simulink model "qr8x8"  (R2018b)
settings: Solver=VariableStepAuto  StartTime=0.0  StopTime=10.0  RelTol=1e-3
libraries: hdlsllib x71, simulink x16, dspmathops x1
(part 1 of 2)
settings Model: Creator=lbai  LastModifiedBy=lbai

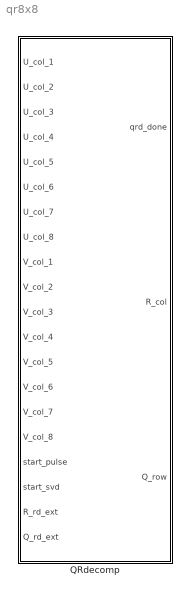
== system qr8x8 ==
  QRdecomp : Subsystem

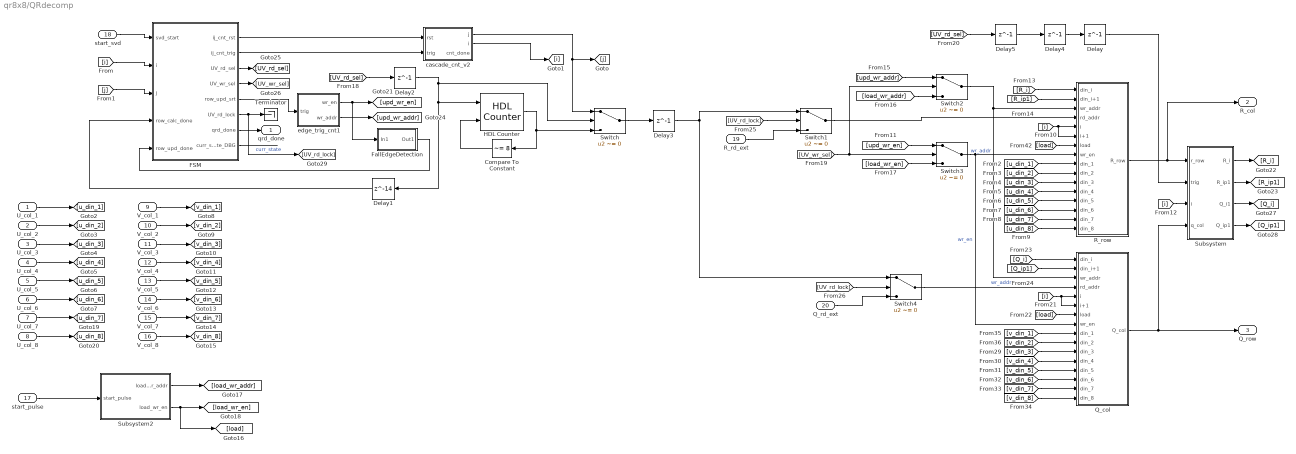
== system qr8x8/QRdecomp ==
  U_col_1 : Inport
  U_col_2 : Inport  Port=2
  U_col_3 : Inport  Port=3
  U_col_4 : Inport  Port=4
  U_col_5 : Inport  Port=5
  U_col_6 : Inport  Port=6
  U_col_7 : Inport  Port=7
  U_col_8 : Inport  Port=8
  V_col_1 : Inport  Port=9
  V_col_2 : Inport  Port=10
  V_col_3 : Inport  Port=11
  V_col_4 : Inport  Port=12
  V_col_5 : Inport  Port=13
  V_col_6 : Inport  Port=14
  V_col_7 : Inport  Port=15
  V_col_8 : Inport  Port=16
  start_pulse : Inport  Port=17
  start_svd : Inport  Port=18
  R_rd_ext : Inport  Port=19
  Q_rd_ext : Inport  Port=20
  Compare To Constant : simulink/Logic and Bit Operations/Compare To Constant  relop=~=  const=8  OutDataTypeStr=boolean
  Delay{,2..5} (5 alike) : Delay  DelayLength=1
  Delay1 : Delay  DelayLength=14
  FSM : MATLAB Function  TreatAsAtomicUnit=on
  FallEdgeDetection : Subsystem
  HDL Counter : hdlsllib/Sources/HDL Counter  CountType=Count limited  CountInit=1  CountStep=1  CountMax=8  CountFromType=Initial value  CountFrom=1  CountResetPort=on  CountLoadPort=off  CountEnbPort=on  CountDirPort=off  CountDataType=Unsigned  CountWordLen=4  CountFracLen=0  CountSampTime=1
      settings: SourceProductBaseCode=HD
  Q_col : Subsystem
  R_row : Subsystem
  Subsystem : Subsystem
  Subsystem2 : Subsystem
  Switch{,1..4} (5 alike) : Switch  Criteria=u2 ~= 0
  Terminator : Terminator
  cascade_cnt_v2 : Subsystem
  edge_trig_cnt1 : Subsystem
  qrd_done : Outport
  R_col : Outport  Port=2
  Q_row : Outport  Port=3
  wires:
  Subsystem2/1(load_wr_addr) -> [load_wr_addr]
  Subsystem2/2(load_wr_en) -> [load], [load_wr_en]
  start_pulse/1 -> Subsystem2/1(start_pulse)
  cascade_cnt_v2/2(i) -> [i]
  [j] -> FSM/3(j)
  FSM/8(curr_state_DBG) -> ?  "curr_state"
  [i] -> FSM/2(i)
  Switch/1 -> Delay3/1
  HDL Counter/1 -> Switch/3, Compare To Constant/1
  FSM/2(ij_cnt_trig) -> cascade_cnt_v2/2(trig)
  [UV_rd_sel] -> Delay2/1
  Compare To Constant/1 -> HDL Counter/2
  [u_din_7] -> R_row/15(din_7)
  start_svd/1 -> FSM/1(svd_start)
  [u_din_6] -> R_row/14(din_6)
  [u_din_4] -> R_row/12(din_4)
  [u_din_8] -> R_row/16(din_8)
  [load] -> R_row/7(load)
  [u_din_1] -> R_row/9(din_1)
  cascade_cnt_v2/1(j) -> Switch/1, [j]
  [u_din_3] -> R_row/11(din_3)
  FSM/1(ij_cnt_rst) -> cascade_cnt_v2/1(rst)
  [u_din_5] -> R_row/13(din_5)
  [u_din_2] -> R_row/10(din_2)
  U_col_1/1 -> [u_din_1]
  U_col_2/1 -> [u_din_2]
  U_col_3/1 -> [u_din_3]
  U_col_4/1 -> [u_din_4]
  U_col_5/1 -> [u_din_5]
  U_col_6/1 -> [u_din_6]
  U_col_7/1 -> [u_din_7]
  U_col_8/1 -> [u_din_8]
  V_col_8/1 -> [v_din_8]
  V_col_7/1 -> [v_din_7]
  V_col_3/1 -> [v_din_3]
  V_col_1/1 -> [v_din_1]
  V_col_4/1 -> [v_din_4]
  V_col_5/1 -> [v_din_5]
  V_col_6/1 -> [v_din_6]
  V_col_2/1 -> [v_din_2]
  [load_wr_en] -> Switch3/3
  [load_wr_addr] -> Switch2/3
  Switch2/1 -> Q_col/3(wr_addr), R_row/3(wr_addr)  "wr_addr"
  Switch3/1 -> Q_col/8(wr_en), R_row/8(wr_en)  "wr_en"
  [UV_wr_sel] -> Switch2/2, Switch3/2
  Switch1/1 -> R_row/4(rd_addr)
  Delay4/1 -> Delay/1
  [i] -> R_row/6(i+1), R_row/5(i)
  [R_i] -> R_row/1(din_i)
  [R_ip1] -> R_row/2(din_i+1)
  R_row/1(R_row) -> R_col/1, Subsystem/1(r_row)
  Delay/1 -> Subsystem/2(trig)
  [i] -> Subsystem/3(i)
  Subsystem/1(R_i) -> [R_i]
  Subsystem/2(R_ip1) -> [R_ip1]
  edge_trig_cnt1/1(wr_en) -> [upd_wr_en], FallEdgeDetection/1(In1)
  FSM/5(row_upd_srt) -> edge_trig_cnt1/1(trig)
  edge_trig_cnt1/2(wr_addr) -> [upd_wr_addr]
  Delay1/1 -> FSM/4(row_calc_done)
  FallEdgeDetection/1(Out1) -> FSM/5(row_upd_done)
  FSM/3(UV_rd_sel) -> [UV_rd_sel]
  FSM/4(UV_wr_sel) -> [UV_wr_sel]
  [upd_wr_en] -> Switch3/1
  [upd_wr_addr] -> Switch2/1
  Delay2/1 -> Delay1/1, HDL Counter/1, Switch/2
  [UV_rd_sel] -> Delay5/1
  Delay5/1 -> Delay4/1
  [v_din_2] -> Q_col/10(din_2)
  [v_din_5] -> Q_col/13(din_5)
  [v_din_3] -> Q_col/11(din_3)
  [v_din_1] -> Q_col/9(din_1)
  [v_din_8] -> Q_col/16(din_8)
  [v_din_4] -> Q_col/12(din_4)
  [v_din_6] -> Q_col/14(din_6)
  [v_din_7] -> Q_col/15(din_7)
  [i] -> Q_col/6(i+1), Q_col/5(i)
  [load] -> Q_col/7(load)
  Q_col/1(Q_col) -> Q_row/1, Subsystem/4(q_col)
  [Q_i] -> Q_col/1(din_i)
  [Q_ip1] -> Q_col/2(din_i+1)
  Subsystem/3(Q_i1) -> [Q_i]
  Subsystem/4(Q_ip1) -> [Q_ip1]
  FSM/7(qrd_done) -> qrd_done/1
  FSM/6(UV_rd_lock) -> Terminator/1, [UV_rd_lock]
  [UV_rd_lock] -> Switch1/2
  [UV_rd_lock] -> Switch4/2
  R_rd_ext/1 -> Switch1/3
  Q_rd_ext/1 -> Switch4/3
  Switch4/1 -> Q_col/4(rd_addr)  "wr_addr"
  Delay3/1 -> Switch4/1, Switch1/1

== system qr8x8/QRdecomp/FallEdgeDetection ==
  In1 : Inport
  Delay : Delay  DelayLength=1
  Logical Operator : Logic  AllPortsSameDT=off  OutDataTypeStr=boolean
  Logical Operator2 : Logic  Operator=NOT  AllPortsSameDT=off  OutDataTypeStr=boolean
  Out1 : Outport
  wires:
  In1/1 -> Logical Operator2/1, Delay/1
  Delay/1 -> Logical Operator/1
  Logical Operator/1 -> Out1/1
  Logical Operator2/1 -> Logical Operator/2

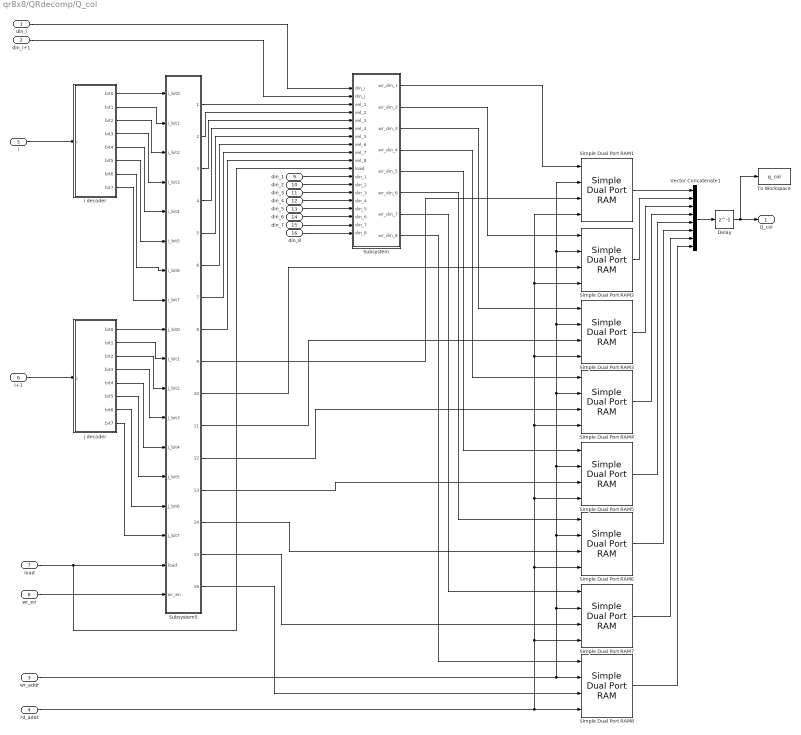
== system qr8x8/QRdecomp/Q_col ==
  din_i : Inport
  din_i+1 : Inport  Port=2
  wr_addr : Inport  Port=3
  rd_addr : Inport  Port=4
  i : Inport  Port=5
  i+1 : Inport  Port=6
  load : Inport  Port=7
  wr_en : Inport  Port=8
  din_1 : Inport  Port=9
  din_2 : Inport  Port=10
  din_3 : Inport  Port=11
  din_4 : Inport  Port=12
  din_5 : Inport  Port=13
  din_6 : Inport  Port=14
  din_7 : Inport  Port=15
  din_8 : Inport  Port=16
  Delay : Delay  DelayLength=1
  Simple Dual Port RAM{1..8} (8 alike) : hdlsllib/HDL RAMs/Simple Dual Port RAM  ram_size=4
      settings: SourceProductName=HDL Coder  SourceProductBaseCode=HD
  Subsystem : Subsystem
  Subsystem5 : Subsystem
  To Workspace : ToWorkspace  VariableName=q_col  SaveFormat=Timeseries  SampleTime=-1
  Vector Concatenate1 : Concatenate  NumInputs=8
  i decoder : MATLAB Function  TreatAsAtomicUnit=on
  j decoder : MATLAB Function  TreatAsAtomicUnit=on
  Q_col : Outport
  wires:
  i+1/1 -> j decoder/1(j)
  Delay/1 -> Q_col/1, To Workspace/1
  Vector Concatenate1/1 -> Delay/1
  Simple Dual Port RAM3/1 -> Vector Concatenate1/3
  Simple Dual Port RAM4/1 -> Vector Concatenate1/4
  Simple Dual Port RAM5/1 -> Vector Concatenate1/5
  Simple Dual Port RAM6/1 -> Vector Concatenate1/6
  Simple Dual Port RAM7/1 -> Vector Concatenate1/7
  Simple Dual Port RAM8/1 -> Vector Concatenate1/8
  i/1 -> i decoder/1(i)
  i decoder/1(bit0) -> Subsystem5/1(i_bit0)
  j decoder/1(bit0) -> Subsystem5/9(j_bit0)
  i decoder/2(bit1) -> Subsystem5/2(i_bit1)
  i decoder/3(bit2) -> Subsystem5/3(i_bit2)
  i decoder/4(bit3) -> Subsystem5/4(i_bit3)
  i decoder/5(bit4) -> Subsystem5/5(i_bit4)
  i decoder/6(bit5) -> Subsystem5/6(i_bit5)
  i decoder/7(bit6) -> Subsystem5/7(i_bit6)
  i decoder/8(bit7) -> Subsystem5/8(i_bit7)
  j decoder/2(bit1) -> Subsystem5/10(j_bit1)
  j decoder/3(bit2) -> Subsystem5/11(j_bit2)
  j decoder/4(bit3) -> Subsystem5/12(j_bit3)
  j decoder/5(bit4) -> Subsystem5/13(j_bit4)
  j decoder/6(bit5) -> Subsystem5/14(j_bit5)
  j decoder/7(bit6) -> Subsystem5/15(j_bit6)
  j decoder/8(bit7) -> Subsystem5/16(j_bit7)
  Subsystem5/9(wr_en_0) -> Simple Dual Port RAM1/3
  Subsystem5/10(wr_en_1) -> Simple Dual Port RAM2/3
  Subsystem5/11(wr_en_2) -> Simple Dual Port RAM3/3
  Subsystem5/12(wr_en_3) -> Simple Dual Port RAM4/3
  Subsystem5/13(wr_en_4) -> Simple Dual Port RAM5/3
  Subsystem5/14(wr_en_5) -> Simple Dual Port RAM6/3
  Subsystem5/15(wr_en_6) -> Simple Dual Port RAM7/3
  Subsystem5/16(wr_en_7) -> Simple Dual Port RAM8/3
  Subsystem5/8(wr_sel_7) -> Subsystem/10(sel_8)
  Subsystem5/7(wr_sel_6) -> Subsystem/9(sel_7)
  Subsystem5/6(wr_sel_5) -> Subsystem/8(sel_6)
  Subsystem5/5(wr_sel_4) -> Subsystem/7(sel_5)
  Subsystem5/4(wr_sel_3) -> Subsystem/6(sel_4)
  Subsystem5/3(wr_sel_2) -> Subsystem/5(sel_3)
  Subsystem5/2(wr_sel_1) -> Subsystem/4(sel_2)
  Subsystem5/1(wr_sel_0) -> Subsystem/3(sel_1)
  din_i/1 -> Subsystem/1(din_i)
  din_i+1/1 -> Subsystem/2("din_j ")
  wr_addr/1 -> Simple Dual Port RAM8/2, Simple Dual Port RAM7/2, Simple Dual Port RAM6/2, Simple Dual Port RAM5/2, Simple Dual Port RAM4/2, Simple Dual Port RAM3/2, Simple Dual Port RAM2/2, Simple Dual Port RAM1/2
  rd_addr/1 -> Simple Dual Port RAM8/4, Simple Dual Port RAM7/4, Simple Dual Port RAM6/4, Simple Dual Port RAM5/4, Simple Dual Port RAM4/4, Simple Dual Port RAM3/4, Simple Dual Port RAM2/4, Simple Dual Port RAM1/4
  Subsystem/1(wr_din_1) -> Simple Dual Port RAM1/1
  Subsystem/2(wr_din_2) -> Simple Dual Port RAM2/1
  Subsystem/3(wr_din_3) -> Simple Dual Port RAM3/1
  Subsystem/4(wr_din_4) -> Simple Dual Port RAM4/1
  Subsystem/5(wr_din_5) -> Simple Dual Port RAM5/1
  Subsystem/6(wr_din_6) -> Simple Dual Port RAM6/1
  Subsystem/7(wr_din_7) -> Simple Dual Port RAM7/1
  Subsystem/8(wr_din_8) -> Simple Dual Port RAM8/1
  wr_en/1 -> Subsystem5/18(wr_en)
  load/1 -> Subsystem/11(load), Subsystem5/17(load)
  din_1/1 -> Subsystem/12(din_1)
  din_2/1 -> Subsystem/13(din_2)
  din_3/1 -> Subsystem/14(din_3)
  din_4/1 -> Subsystem/15(din_4)
  din_5/1 -> Subsystem/16(din_5)
  din_8/1 -> Subsystem/19(din_8)
  din_7/1 -> Subsystem/18(din_7)
  din_6/1 -> Subsystem/17(din_6)
  Simple Dual Port RAM1/1 -> Vector Concatenate1/1
  Simple Dual Port RAM2/1 -> Vector Concatenate1/2

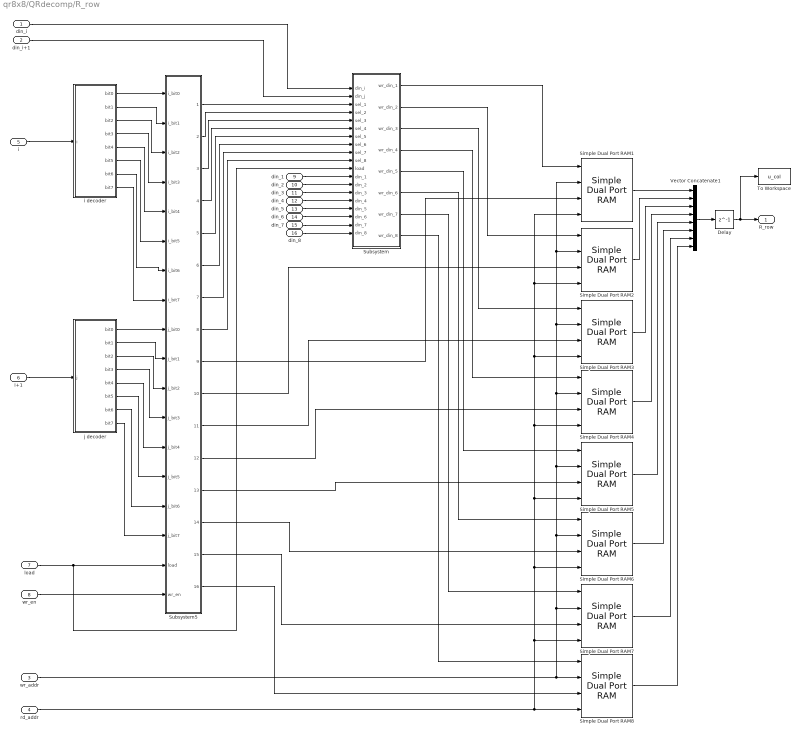
== system qr8x8/QRdecomp/R_row ==
  din_i : Inport
  din_i+1 : Inport  Port=2
  wr_addr : Inport  Port=3
  rd_addr : Inport  Port=4
  i : Inport  Port=5
  i+1 : Inport  Port=6
  load : Inport  Port=7
  wr_en : Inport  Port=8
  din_1 : Inport  Port=9
  din_2 : Inport  Port=10
  din_3 : Inport  Port=11
  din_4 : Inport  Port=12
  din_5 : Inport  Port=13
  din_6 : Inport  Port=14
  din_7 : Inport  Port=15
  din_8 : Inport  Port=16
  Delay : Delay  DelayLength=1
  Simple Dual Port RAM{1..8} (8 alike) : hdlsllib/HDL RAMs/Simple Dual Port RAM  ram_size=4
      settings: SourceProductName=HDL Coder  SourceProductBaseCode=HD
  Subsystem : Subsystem
  Subsystem5 : Subsystem
  To Workspace : ToWorkspace  VariableName=u_col  SaveFormat=Timeseries  SampleTime=-1
  Vector Concatenate1 : Concatenate  NumInputs=8
  i decoder : MATLAB Function  TreatAsAtomicUnit=on
  j decoder : MATLAB Function  TreatAsAtomicUnit=on
  R_row : Outport
  wires:
  Simple Dual Port RAM2/1 -> Vector Concatenate1/2
  Simple Dual Port RAM1/1 -> Vector Concatenate1/1
  din_6/1 -> Subsystem/17(din_6)
  din_7/1 -> Subsystem/18(din_7)
  din_8/1 -> Subsystem/19(din_8)
  din_5/1 -> Subsystem/16(din_5)
  din_4/1 -> Subsystem/15(din_4)
  din_3/1 -> Subsystem/14(din_3)
  din_2/1 -> Subsystem/13(din_2)
  din_1/1 -> Subsystem/12(din_1)
  load/1 -> Subsystem5/17(load), Subsystem/11(load)
  wr_en/1 -> Subsystem5/18(wr_en)
  Subsystem/8(wr_din_8) -> Simple Dual Port RAM8/1
  Subsystem/7(wr_din_7) -> Simple Dual Port RAM7/1
  Subsystem/6(wr_din_6) -> Simple Dual Port RAM6/1
  Subsystem/5(wr_din_5) -> Simple Dual Port RAM5/1
  Subsystem/4(wr_din_4) -> Simple Dual Port RAM4/1
  Subsystem/3(wr_din_3) -> Simple Dual Port RAM3/1
  Subsystem/2(wr_din_2) -> Simple Dual Port RAM2/1
  Subsystem/1(wr_din_1) -> Simple Dual Port RAM1/1
  rd_addr/1 -> Simple Dual Port RAM1/4, Simple Dual Port RAM2/4, Simple Dual Port RAM3/4, Simple Dual Port RAM4/4, Simple Dual Port RAM5/4, Simple Dual Port RAM6/4, Simple Dual Port RAM7/4, Simple Dual Port RAM8/4
  wr_addr/1 -> Simple Dual Port RAM1/2, Simple Dual Port RAM2/2, Simple Dual Port RAM3/2, Simple Dual Port RAM4/2, Simple Dual Port RAM5/2, Simple Dual Port RAM6/2, Simple Dual Port RAM7/2, Simple Dual Port RAM8/2
  din_i+1/1 -> Subsystem/2("din_j ")
  din_i/1 -> Subsystem/1(din_i)
  Subsystem5/1(wr_sel_0) -> Subsystem/3(sel_1)
  Subsystem5/2(wr_sel_1) -> Subsystem/4(sel_2)
  Subsystem5/3(wr_sel_2) -> Subsystem/5(sel_3)
  Subsystem5/4(wr_sel_3) -> Subsystem/6(sel_4)
  Subsystem5/5(wr_sel_4) -> Subsystem/7(sel_5)
  Subsystem5/6(wr_sel_5) -> Subsystem/8(sel_6)
  Subsystem5/7(wr_sel_6) -> Subsystem/9(sel_7)
  Subsystem5/8(wr_sel_7) -> Subsystem/10(sel_8)
  Subsystem5/16(wr_en_7) -> Simple Dual Port RAM8/3
  Subsystem5/15(wr_en_6) -> Simple Dual Port RAM7/3
  Subsystem5/14(wr_en_5) -> Simple Dual Port RAM6/3
  Subsystem5/13(wr_en_4) -> Simple Dual Port RAM5/3
  Subsystem5/12(wr_en_3) -> Simple Dual Port RAM4/3
  Subsystem5/11(wr_en_2) -> Simple Dual Port RAM3/3
  Subsystem5/10(wr_en_1) -> Simple Dual Port RAM2/3
  Subsystem5/9(wr_en_0) -> Simple Dual Port RAM1/3
  j decoder/8(bit7) -> Subsystem5/16(j_bit7)
  j decoder/7(bit6) -> Subsystem5/15(j_bit6)
  j decoder/6(bit5) -> Subsystem5/14(j_bit5)
  j decoder/5(bit4) -> Subsystem5/13(j_bit4)
  j decoder/4(bit3) -> Subsystem5/12(j_bit3)
  j decoder/3(bit2) -> Subsystem5/11(j_bit2)
  j decoder/2(bit1) -> Subsystem5/10(j_bit1)
  i decoder/8(bit7) -> Subsystem5/8(i_bit7)
  i decoder/7(bit6) -> Subsystem5/7(i_bit6)
  i decoder/6(bit5) -> Subsystem5/6(i_bit5)
  i decoder/5(bit4) -> Subsystem5/5(i_bit4)
  i decoder/4(bit3) -> Subsystem5/4(i_bit3)
  i decoder/3(bit2) -> Subsystem5/3(i_bit2)
  i decoder/2(bit1) -> Subsystem5/2(i_bit1)
  j decoder/1(bit0) -> Subsystem5/9(j_bit0)
  i decoder/1(bit0) -> Subsystem5/1(i_bit0)
  i/1 -> i decoder/1(i)
  Simple Dual Port RAM8/1 -> Vector Concatenate1/8
  Simple Dual Port RAM7/1 -> Vector Concatenate1/7
  Simple Dual Port RAM6/1 -> Vector Concatenate1/6
  Simple Dual Port RAM5/1 -> Vector Concatenate1/5
  Simple Dual Port RAM4/1 -> Vector Concatenate1/4
  Simple Dual Port RAM3/1 -> Vector Concatenate1/3
  Vector Concatenate1/1 -> Delay/1
  Delay/1 -> To Workspace/1, R_row/1
  i+1/1 -> j decoder/1(j)

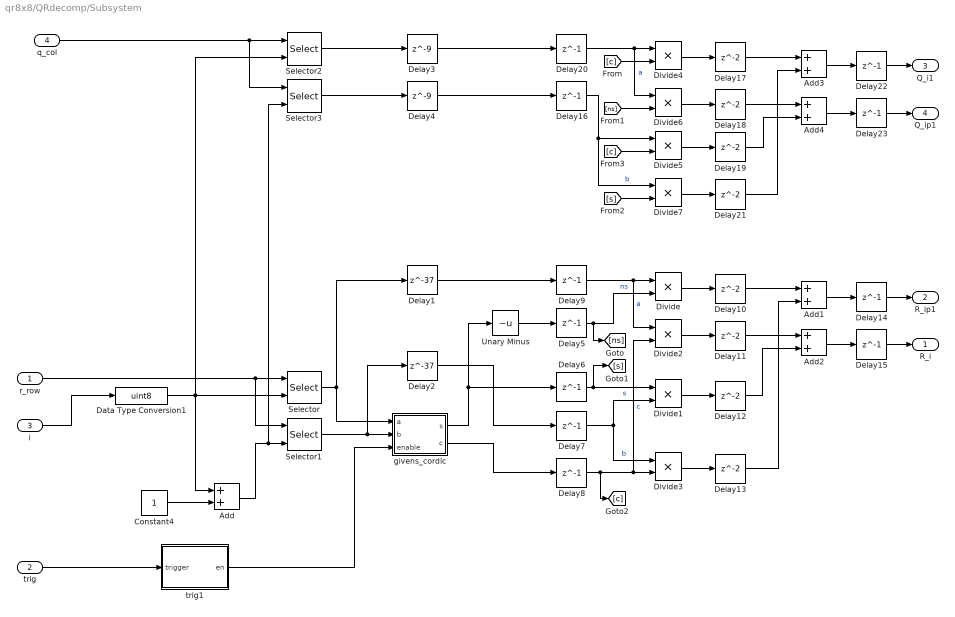
== system qr8x8/QRdecomp/Subsystem ==
  r_row : Inport
  trig : Inport  Port=2
  i : Inport  Port=3
  q_col : Inport  Port=4
  Add : Sum  OutDataTypeStr=Inherit: Same as first input
  Add1 : Sum
  Add2 : Sum
  Add3 : Sum  OutDataTypeStr=fixdt(1,32,30)
  Add4 : Sum  OutDataTypeStr=fixdt(1,32,30)
  Constant4 : Constant  OutDataTypeStr=fixdt(0,1,0)  SampleTime=-1
  Data Type Conversion1 : DataTypeConversion  OutDataTypeStr=uint8
  Delay1 : Delay  DelayLength=37
  Delay{10..13,17..19,21} (8 alike) : Delay
  Delay{5..9,14..16,20,22..23} (11 alike) : Delay  DelayLength=1
  Delay2 : Delay  DelayLength=37
  Delay3 : Delay  DelayLength=9
  Delay4 : Delay  DelayLength=9
  Divide{,1..3} (4 alike) : Product  Inputs=**  OutDataTypeStr=fixdt(1,32,25)  SaturateOnIntegerOverflow=on  RndMeth=Zero
  Divide{4..7} (4 alike) : Product  Inputs=**  OutDataTypeStr=fixdt(1,32,30)  SaturateOnIntegerOverflow=on  RndMeth=Zero
  Selector{,1..3} (4 alike) : Selector  InputPortWidth=8  IndexOptions=Index vector (port)  Indices=[1 3]  OutputSizes=1
  Unary Minus : UnaryMinus
  givens_cordic : Subsystem
  trig1 : Subsystem
  R_i : Outport
  R_ip1 : Outport  Port=2
  Q_i1 : Outport  Port=3
  Q_ip1 : Outport  Port=4
  wires:
  Add1/1 -> Delay14/1
  Delay9/1 -> Divide2/1, Divide/1  "a"
  Unary Minus/1 -> Delay5/1
  Delay8/1 -> [c], Divide2/2, Divide3/2  "c"
  givens_cordic/1(s) -> Unary Minus/1, Delay6/1
  Selector/1 -> givens_cordic/1(a), Delay1/1
  Constant4/1 -> Add/2
  Divide2/1 -> Delay11/1
  Selector1/1 -> givens_cordic/2(b), Delay2/1
  Delay7/1 -> Divide3/1, Divide1/2  "b"
  Divide3/1 -> Delay13/1
  i/1 -> Data Type Conversion1/1
  givens_cordic/2(c) -> Delay8/1
  Delay11/1 -> Add2/1
  trig1/1(en) -> givens_cordic/3(enable)
  r_row/1 -> Selector/1, Selector1/1
  Delay5/1 -> [ns], Divide/2  "ns"
  Delay2/1 -> Delay7/1
  Delay10/1 -> Add1/1
  Delay1/1 -> Delay9/1
  Add2/1 -> Delay15/1
  Delay13/1 -> Add1/2
  Delay12/1 -> Add2/2
  Divide1/1 -> Delay12/1
  Divide/1 -> Delay10/1
  Delay6/1 -> Divide1/1, [s]  "s"
  trig/1 -> trig1/1(trigger)
  Add/1 -> Selector3/2, Selector1/2
  Data Type Conversion1/1 -> Selector2/2, Add/1, Selector/2
  Delay15/1 -> R_i/1
  Delay14/1 -> R_ip1/1
  q_col/1 -> Selector3/1, Selector2/1
  Selector2/1 -> Delay3/1
  Selector3/1 -> Delay4/1
  Delay3/1 -> Delay20/1
  Delay4/1 -> Delay16/1
  Delay20/1 -> Divide6/1, Divide4/1  "a"
  [c] -> Divide4/2
  Delay19/1 -> Add4/2
  Delay21/1 -> Add3/2
  Add4/1 -> Delay23/1
  Delay17/1 -> Add3/1
  Delay18/1 -> Add4/1
  Add3/1 -> Delay22/1
  Divide4/1 -> Delay17/1
  Divide6/1 -> Delay18/1
  Divide5/1 -> Delay19/1
  Divide7/1 -> Delay21/1
  Delay16/1 -> Divide5/1, Divide7/1  "b"
  [s] -> Divide7/2
  [ns] -> Divide6/2
  [c] -> Divide5/2
  Delay22/1 -> Q_i1/1
  Delay23/1 -> Q_ip1/1

== system qr8x8/QRdecomp/Subsystem2 ==
  start_pulse : Inport
  Compare To Constant2 : simulink/Logic and Bit Operations/Compare To Constant  relop===  const=8  OutDataTypeStr=boolean
  Compare To Constant3 : simulink/Logic and Bit Operations/Compare To Constant  relop===  const=0  OutDataTypeStr=boolean
  Constant : Constant  OutDataTypeStr=boolean  SampleTime=-1
  Delay1 : Delay  DelayLength=1
  Delay3 : Delay
  Enabled Resettable Delay : Delay  DelayLength=1  ExternalReset=Level
      settings: InputPortMap=u0,r5
  HDL Counter : hdlsllib/Sources/HDL Counter  CountType=Count limited  CountInit=0  CountStep=1  CountMax=8  CountFromType=Initial value  CountFrom=0  CountResetPort=on  CountLoadPort=off  CountEnbPort=on  CountDirPort=off  CountDataType=Unsigned  CountWordLen=4  CountFracLen=0  CountSampTime=1
      settings: SourceProductBaseCode=HD
  Switch : Switch  Criteria=u2 ~= 0
  load_wr_addr : Outport
  load_wr_en : Outport  Port=2
  wires:
  Compare To Constant3/1 -> HDL Counter/1
  Enabled Resettable Delay/1 -> Delay3/1, HDL Counter/2, Compare To Constant3/1, Switch/3
  Compare To Constant2/1 -> Enabled Resettable Delay/2
  HDL Counter/1 -> Delay1/1, Compare To Constant2/1
  Delay3/1 -> load_wr_en/1
  Constant/1 -> Switch/1
  Switch/1 -> Enabled Resettable Delay/1
  start_pulse/1 -> Switch/2
  Delay1/1 -> load_wr_addr/1

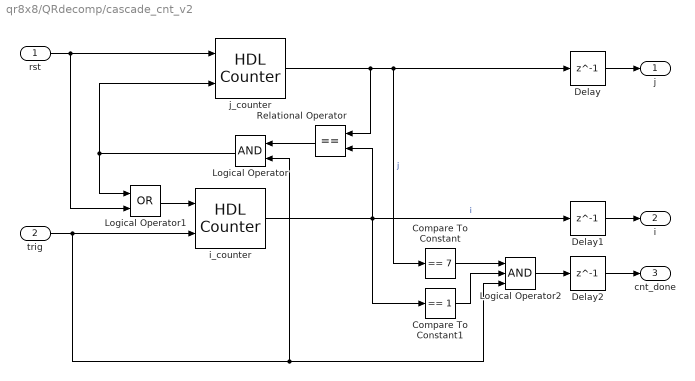
== system qr8x8/QRdecomp/cascade_cnt_v2 ==
  rst : Inport
  trig : Inport  Port=2
  Compare To Constant : simulink/Logic and Bit Operations/Compare To Constant  relop===  const=7  OutDataTypeStr=boolean
  Compare To Constant1 : simulink/Logic and Bit Operations/Compare To Constant  relop===  const=1  OutDataTypeStr=boolean
  Delay : Delay  DelayLength=1
  Delay1 : Delay  DelayLength=1
  Delay2 : Delay  DelayLength=1
  Logical Operator : Logic  AllPortsSameDT=off  OutDataTypeStr=boolean
  Logical Operator1 : Logic  Operator=OR  AllPortsSameDT=off  OutDataTypeStr=boolean
  Logical Operator2 : Logic  Inputs=3  AllPortsSameDT=off  OutDataTypeStr=boolean
  Relational Operator : RelationalOperator  Operator===  OutDataTypeStr=boolean  RndMeth=Nearest
  i_counter : hdlsllib/Sources/HDL Counter  CountType=Count limited  CountInit=7  CountStep=-1  CountMax=1  CountFromType=Initial value  CountFrom=7  CountResetPort=on  CountLoadPort=off  CountEnbPort=on  CountDirPort=off  CountDataType=Unsigned  CountWordLen=4  CountFracLen=0  CountSampTime=1
      settings: SourceProductBaseCode=HD
  j_counter : hdlsllib/Sources/HDL Counter  CountType=Count limited  CountInit=1  CountStep=1  CountMax=7  CountFromType=Initial value  CountFrom=1  CountResetPort=on  CountLoadPort=off  CountEnbPort=on  CountDirPort=off  CountDataType=Unsigned  CountWordLen=4  CountFracLen=0  CountSampTime=1
      settings: SourceProductBaseCode=HD
  j : Outport
  i : Outport  Port=2
  cnt_done : Outport  Port=3
  wires:
  trig/1 -> i_counter/2, Logical Operator/2, Logical Operator2/3
  rst/1 -> Logical Operator1/2, j_counter/1
  j_counter/1 -> Delay/1, Compare To Constant/1, Relational Operator/1  "j"
  i_counter/1 -> Delay1/1, Compare To Constant1/1, Relational Operator/2  "i"
  Relational Operator/1 -> Logical Operator/1
  Logical Operator/1 -> Logical Operator1/1, j_counter/2
  Delay/1 -> j/1
  Delay1/1 -> i/1
  Logical Operator1/1 -> i_counter/1
  Compare To Constant/1 -> Logical Operator2/1
  Compare To Constant1/1 -> Logical Operator2/2
  Logical Operator2/1 -> Delay2/1
  Delay2/1 -> cnt_done/1

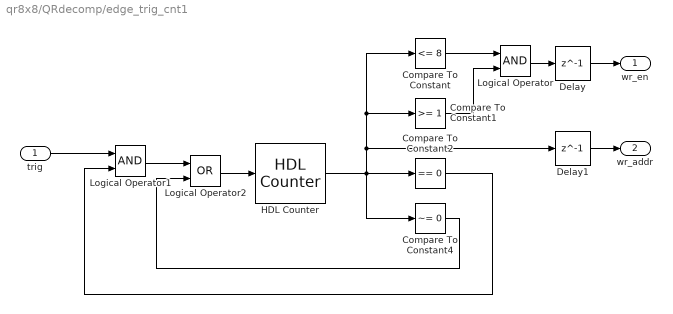
== system qr8x8/QRdecomp/edge_trig_cnt1 ==
  trig : Inport
  Compare To Constant : simulink/Logic and Bit Operations/Compare To Constant  relop=<=  const=8  OutDataTypeStr=boolean
  Compare To Constant1 : simulink/Logic and Bit Operations/Compare To Constant  relop=>=  const=1  OutDataTypeStr=boolean
  Compare To Constant2 : simulink/Logic and Bit Operations/Compare To Constant  relop===  const=0  OutDataTypeStr=boolean
  Compare To Constant4 : simulink/Logic and Bit Operations/Compare To Constant  relop=~=  const=0  OutDataTypeStr=boolean
  Delay : Delay  DelayLength=1
  Delay1 : Delay  DelayLength=1
  HDL Counter : hdlsllib/Sources/HDL Counter  CountType=Count limited  CountInit=0  CountStep=1  CountMax=9  CountFromType=Initial value  CountFrom=0  CountResetPort=off  CountLoadPort=off  CountEnbPort=on  CountDirPort=off  CountDataType=Unsigned  CountWordLen=4  CountFracLen=0  CountSampTime=1
      settings: SourceProductBaseCode=HD
  Logical Operator : Logic  AllPortsSameDT=off  OutDataTypeStr=boolean
  Logical Operator1 : Logic  AllPortsSameDT=off  OutDataTypeStr=boolean
  Logical Operator2 : Logic  Operator=OR  AllPortsSameDT=off  OutDataTypeStr=boolean
  wr_en : Outport
  wr_addr : Outport  Port=2
  wires:
  Delay/1 -> wr_en/1
  Logical Operator2/1 -> HDL Counter/1
  Logical Operator/1 -> Delay/1
  Compare To Constant2/1 -> Logical Operator1/2
  Compare To Constant1/1 -> Logical Operator/2
  trig/1 -> Logical Operator1/1
  Compare To Constant/1 -> Logical Operator/1
  HDL Counter/1 -> Compare To Constant2/1, Compare To Constant4/1, Delay1/1, Compare To Constant1/1, Compare To Constant/1
  Logical Operator1/1 -> Logical Operator2/1
  Compare To Constant4/1 -> Logical Operator2/2
  Delay1/1 -> wr_addr/1

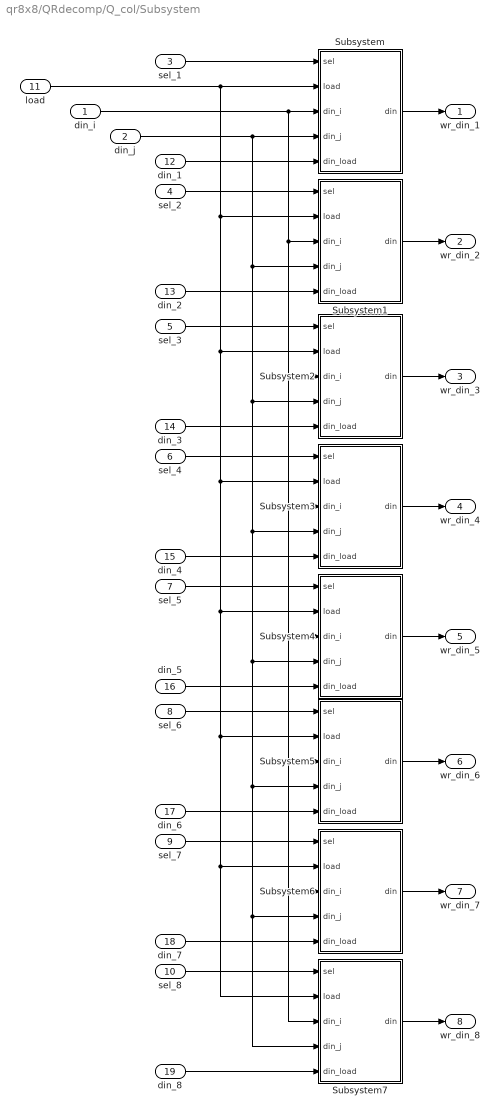
== system qr8x8/QRdecomp/Q_col/Subsystem ==
  din_i : Inport
  "din_j " : Inport  Port=2
  sel_1 : Inport  Port=3
  sel_2 : Inport  Port=4
  sel_3 : Inport  Port=5
  sel_4 : Inport  Port=6
  sel_5 : Inport  Port=7
  sel_6 : Inport  Port=8
  sel_7 : Inport  Port=9
  sel_8 : Inport  Port=10
  load : Inport  Port=11
  din_1 : Inport  Port=12
  din_2 : Inport  Port=13
  din_3 : Inport  Port=14
  din_4 : Inport  Port=15
  din_5 : Inport  Port=16
  din_6 : Inport  Port=17
  din_7 : Inport  Port=18
  din_8 : Inport  Port=19
  Subsystem : Subsystem
  Subsystem1 : Subsystem
  Subsystem2 : Subsystem
  Subsystem3 : Subsystem
  Subsystem4 : Subsystem
  Subsystem5 : Subsystem
  Subsystem6 : Subsystem
  Subsystem7 : Subsystem
  wr_din_1 : Outport
  wr_din_2 : Outport  Port=2
  wr_din_3 : Outport  Port=3
  wr_din_4 : Outport  Port=4
  wr_din_5 : Outport  Port=5
  wr_din_6 : Outport  Port=6
  wr_din_7 : Outport  Port=7
  wr_din_8 : Outport  Port=8
  wires:
  sel_1/1 -> Subsystem/1(sel)
  Subsystem/1(din) -> wr_din_1/1
  "din_j "/1 -> Subsystem/4("din_j "), Subsystem1/4("din_j "), Subsystem2/4("din_j "), Subsystem3/4("din_j "), Subsystem4/4("din_j "), Subsystem5/4("din_j "), Subsystem7/4("din_j "), Subsystem6/4("din_j ")
  Subsystem1/1(din) -> wr_din_2/1
  Subsystem2/1(din) -> wr_din_3/1
  Subsystem3/1(din) -> wr_din_4/1
  Subsystem4/1(din) -> wr_din_5/1
  Subsystem5/1(din) -> wr_din_6/1
  Subsystem6/1(din) -> wr_din_7/1
  Subsystem7/1(din) -> wr_din_8/1
  sel_2/1 -> Subsystem1/1(sel)
  sel_3/1 -> Subsystem2/1(sel)
  sel_4/1 -> Subsystem3/1(sel)
  sel_5/1 -> Subsystem4/1(sel)
  sel_8/1 -> Subsystem7/1(sel)
  load/1 -> Subsystem7/2(load), Subsystem6/2(load), Subsystem5/2(load), Subsystem4/2(load), Subsystem3/2(load), Subsystem2/2(load), Subsystem1/2(load), Subsystem/2(load)
  din_1/1 -> Subsystem/5(din_load)
  din_2/1 -> Subsystem1/5(din_load)
  din_i/1 -> Subsystem/3(din_i), Subsystem2/3(din_i), Subsystem3/3(din_i), Subsystem5/3(din_i), Subsystem7/3(din_i), Subsystem6/3(din_i), Subsystem4/3(din_i), Subsystem1/3(din_i)
  sel_6/1 -> Subsystem5/1(sel)
  sel_7/1 -> Subsystem6/1(sel)
  din_3/1 -> Subsystem2/5(din_load)
  din_4/1 -> Subsystem3/5(din_load)
  din_5/1 -> Subsystem4/5(din_load)
  din_6/1 -> Subsystem5/5(din_load)
  din_7/1 -> Subsystem6/5(din_load)
  din_8/1 -> Subsystem7/5(din_load)

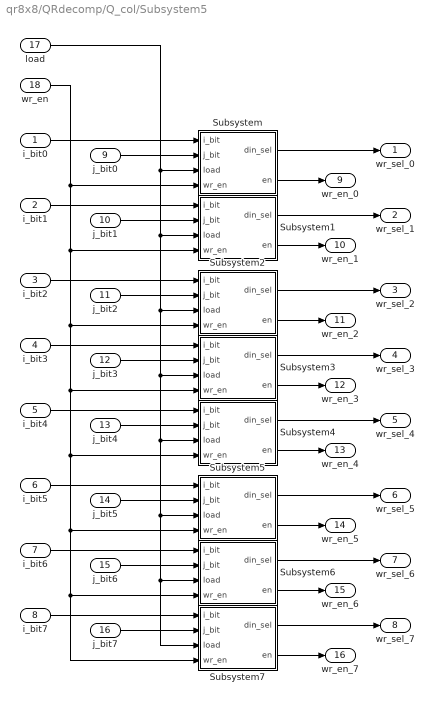
== system qr8x8/QRdecomp/Q_col/Subsystem5 ==
  i_bit0 : Inport
  i_bit1 : Inport  Port=2
  i_bit2 : Inport  Port=3
  i_bit3 : Inport  Port=4
  i_bit4 : Inport  Port=5
  i_bit5 : Inport  Port=6
  i_bit6 : Inport  Port=7
  i_bit7 : Inport  Port=8
  j_bit0 : Inport  Port=9
  j_bit1 : Inport  Port=10
  j_bit2 : Inport  Port=11
  j_bit3 : Inport  Port=12
  j_bit4 : Inport  Port=13
  j_bit5 : Inport  Port=14
  j_bit6 : Inport  Port=15
  j_bit7 : Inport  Port=16
  load : Inport  Port=17
  wr_en : Inport  Port=18
  Subsystem : Subsystem
  Subsystem1 : Subsystem
  Subsystem2 : Subsystem
  Subsystem3 : Subsystem
  Subsystem4 : Subsystem
  Subsystem5 : Subsystem
  Subsystem6 : Subsystem
  Subsystem7 : Subsystem
  wr_sel_0 : Outport
  wr_sel_1 : Outport  Port=2
  wr_sel_2 : Outport  Port=3
  wr_sel_3 : Outport  Port=4
  wr_sel_4 : Outport  Port=5
  wr_sel_5 : Outport  Port=6
  wr_sel_6 : Outport  Port=7
  wr_sel_7 : Outport  Port=8
  wr_en_0 : Outport  Port=9
  wr_en_1 : Outport  Port=10
  wr_en_2 : Outport  Port=11
  wr_en_3 : Outport  Port=12
  wr_en_4 : Outport  Port=13
  wr_en_5 : Outport  Port=14
  wr_en_6 : Outport  Port=15
  wr_en_7 : Outport  Port=16
  wires:
  i_bit1/1 -> Subsystem1/1(i_bit)
  Subsystem4/1(din_sel) -> wr_sel_4/1
  j_bit0/1 -> Subsystem/2(j_bit)
  Subsystem3/2(en) -> wr_en_3/1
  i_bit0/1 -> Subsystem/1(i_bit)
  Subsystem/2(en) -> wr_en_0/1
  i_bit3/1 -> Subsystem3/1(i_bit)
  Subsystem/1(din_sel) -> wr_sel_0/1
  Subsystem2/1(din_sel) -> wr_sel_2/1
  j_bit2/1 -> Subsystem2/2(j_bit)
  j_bit3/1 -> Subsystem3/2(j_bit)
  Subsystem2/2(en) -> wr_en_2/1
  Subsystem3/1(din_sel) -> wr_sel_3/1
  j_bit4/1 -> Subsystem4/2(j_bit)
  Subsystem1/1(din_sel) -> wr_sel_1/1
  Subsystem4/2(en) -> wr_en_4/1
  i_bit4/1 -> Subsystem4/1(i_bit)
  Subsystem1/2(en) -> wr_en_1/1
  i_bit5/1 -> Subsystem5/1(i_bit)
  j_bit5/1 -> Subsystem5/2(j_bit)
  i_bit7/1 -> Subsystem7/1(i_bit)
  j_bit7/1 -> Subsystem7/2(j_bit)
  Subsystem5/1(din_sel) -> wr_sel_5/1
  Subsystem5/2(en) -> wr_en_5/1
  Subsystem6/1(din_sel) -> wr_sel_6/1
  Subsystem6/2(en) -> wr_en_6/1
  Subsystem7/1(din_sel) -> wr_sel_7/1
  Subsystem7/2(en) -> wr_en_7/1
  j_bit1/1 -> Subsystem1/2(j_bit)
  i_bit2/1 -> Subsystem2/1(i_bit)
  i_bit6/1 -> Subsystem6/1(i_bit)
  j_bit6/1 -> Subsystem6/2(j_bit)
  load/1 -> Subsystem1/3(load), Subsystem2/3(load), Subsystem3/3(load), Subsystem4/3(load), Subsystem5/3(load), Subsystem7/3(load), Subsystem6/3(load), Subsystem/3(load)
  wr_en/1 -> Subsystem1/4(wr_en), Subsystem2/4(wr_en), Subsystem3/4(wr_en), Subsystem4/4(wr_en), Subsystem5/4(wr_en), Subsystem7/4(wr_en), Subsystem6/4(wr_en), Subsystem/4(wr_en)

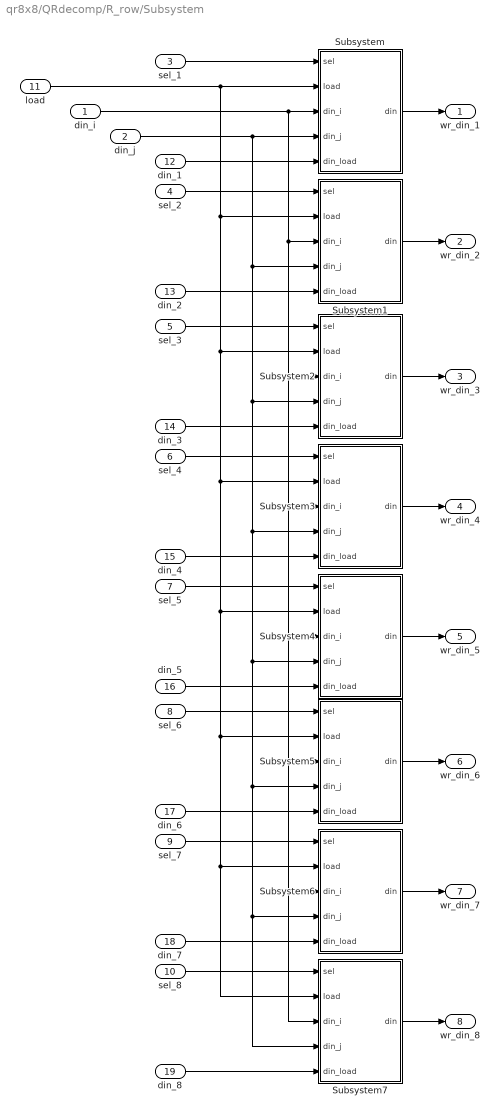
== system qr8x8/QRdecomp/R_row/Subsystem ==
  din_i : Inport
  "din_j " : Inport  Port=2
  sel_1 : Inport  Port=3
  sel_2 : Inport  Port=4
  sel_3 : Inport  Port=5
  sel_4 : Inport  Port=6
  sel_5 : Inport  Port=7
  sel_6 : Inport  Port=8
  sel_7 : Inport  Port=9
  sel_8 : Inport  Port=10
  load : Inport  Port=11
  din_1 : Inport  Port=12
  din_2 : Inport  Port=13
  din_3 : Inport  Port=14
  din_4 : Inport  Port=15
  din_5 : Inport  Port=16
  din_6 : Inport  Port=17
  din_7 : Inport  Port=18
  din_8 : Inport  Port=19
  Subsystem : Subsystem
  Subsystem1 : Subsystem
  Subsystem2 : Subsystem
  Subsystem3 : Subsystem
  Subsystem4 : Subsystem
  Subsystem5 : Subsystem
  Subsystem6 : Subsystem
  Subsystem7 : Subsystem
  wr_din_1 : Outport
  wr_din_2 : Outport  Port=2
  wr_din_3 : Outport  Port=3
  wr_din_4 : Outport  Port=4
  wr_din_5 : Outport  Port=5
  wr_din_6 : Outport  Port=6
  wr_din_7 : Outport  Port=7
  wr_din_8 : Outport  Port=8
  wires:
  din_8/1 -> Subsystem7/5(din_load)
  din_7/1 -> Subsystem6/5(din_load)
  din_6/1 -> Subsystem5/5(din_load)
  din_5/1 -> Subsystem4/5(din_load)
  din_4/1 -> Subsystem3/5(din_load)
  din_3/1 -> Subsystem2/5(din_load)
  sel_7/1 -> Subsystem6/1(sel)
  sel_6/1 -> Subsystem5/1(sel)
  din_i/1 -> Subsystem1/3(din_i), Subsystem4/3(din_i), Subsystem6/3(din_i), Subsystem7/3(din_i), Subsystem5/3(din_i), Subsystem3/3(din_i), Subsystem2/3(din_i), Subsystem/3(din_i)
  din_2/1 -> Subsystem1/5(din_load)
  din_1/1 -> Subsystem/5(din_load)
  load/1 -> Subsystem/2(load), Subsystem1/2(load), Subsystem2/2(load), Subsystem3/2(load), Subsystem4/2(load), Subsystem5/2(load), Subsystem6/2(load), Subsystem7/2(load)
  sel_8/1 -> Subsystem7/1(sel)
  sel_5/1 -> Subsystem4/1(sel)
  sel_4/1 -> Subsystem3/1(sel)
  sel_3/1 -> Subsystem2/1(sel)
  sel_2/1 -> Subsystem1/1(sel)
  Subsystem7/1(din) -> wr_din_8/1
  Subsystem6/1(din) -> wr_din_7/1
  Subsystem5/1(din) -> wr_din_6/1
  Subsystem4/1(din) -> wr_din_5/1
  Subsystem3/1(din) -> wr_din_4/1
  Subsystem2/1(din) -> wr_din_3/1
  Subsystem1/1(din) -> wr_din_2/1
  "din_j "/1 -> Subsystem6/4("din_j "), Subsystem7/4("din_j "), Subsystem5/4("din_j "), Subsystem4/4("din_j "), Subsystem3/4("din_j "), Subsystem2/4("din_j "), Subsystem1/4("din_j "), Subsystem/4("din_j ")
  Subsystem/1(din) -> wr_din_1/1
  sel_1/1 -> Subsystem/1(sel)

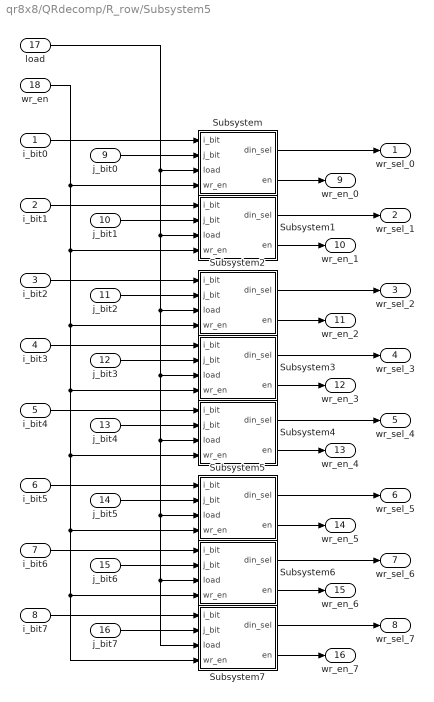
== system qr8x8/QRdecomp/R_row/Subsystem5 ==
  i_bit0 : Inport
  i_bit1 : Inport  Port=2
  i_bit2 : Inport  Port=3
  i_bit3 : Inport  Port=4
  i_bit4 : Inport  Port=5
  i_bit5 : Inport  Port=6
  i_bit6 : Inport  Port=7
  i_bit7 : Inport  Port=8
  j_bit0 : Inport  Port=9
  j_bit1 : Inport  Port=10
  j_bit2 : Inport  Port=11
  j_bit3 : Inport  Port=12
  j_bit4 : Inport  Port=13
  j_bit5 : Inport  Port=14
  j_bit6 : Inport  Port=15
  j_bit7 : Inport  Port=16
  load : Inport  Port=17
  wr_en : Inport  Port=18
  Subsystem : Subsystem
  Subsystem1 : Subsystem
  Subsystem2 : Subsystem
  Subsystem3 : Subsystem
  Subsystem4 : Subsystem
  Subsystem5 : Subsystem
  Subsystem6 : Subsystem
  Subsystem7 : Subsystem
  wr_sel_0 : Outport
  wr_sel_1 : Outport  Port=2
  wr_sel_2 : Outport  Port=3
  wr_sel_3 : Outport  Port=4
  wr_sel_4 : Outport  Port=5
  wr_sel_5 : Outport  Port=6
  wr_sel_6 : Outport  Port=7
  wr_sel_7 : Outport  Port=8
  wr_en_0 : Outport  Port=9
  wr_en_1 : Outport  Port=10
  wr_en_2 : Outport  Port=11
  wr_en_3 : Outport  Port=12
  wr_en_4 : Outport  Port=13
  wr_en_5 : Outport  Port=14
  wr_en_6 : Outport  Port=15
  wr_en_7 : Outport  Port=16
  wires:
  wr_en/1 -> Subsystem/4(wr_en), Subsystem6/4(wr_en), Subsystem7/4(wr_en), Subsystem5/4(wr_en), Subsystem4/4(wr_en), Subsystem3/4(wr_en), Subsystem2/4(wr_en), Subsystem1/4(wr_en)
  load/1 -> Subsystem/3(load), Subsystem6/3(load), Subsystem7/3(load), Subsystem5/3(load), Subsystem4/3(load), Subsystem3/3(load), Subsystem2/3(load), Subsystem1/3(load)
  j_bit6/1 -> Subsystem6/2(j_bit)
  i_bit6/1 -> Subsystem6/1(i_bit)
  i_bit2/1 -> Subsystem2/1(i_bit)
  j_bit1/1 -> Subsystem1/2(j_bit)
  Subsystem7/2(en) -> wr_en_7/1
  Subsystem7/1(din_sel) -> wr_sel_7/1
  Subsystem6/2(en) -> wr_en_6/1
  Subsystem6/1(din_sel) -> wr_sel_6/1
  Subsystem5/2(en) -> wr_en_5/1
  Subsystem5/1(din_sel) -> wr_sel_5/1
  j_bit7/1 -> Subsystem7/2(j_bit)
  i_bit7/1 -> Subsystem7/1(i_bit)
  j_bit5/1 -> Subsystem5/2(j_bit)
  i_bit5/1 -> Subsystem5/1(i_bit)
  Subsystem1/2(en) -> wr_en_1/1
  i_bit4/1 -> Subsystem4/1(i_bit)
  Subsystem4/2(en) -> wr_en_4/1
  Subsystem1/1(din_sel) -> wr_sel_1/1
  j_bit4/1 -> Subsystem4/2(j_bit)
  Subsystem3/1(din_sel) -> wr_sel_3/1
  Subsystem2/2(en) -> wr_en_2/1
  j_bit3/1 -> Subsystem3/2(j_bit)
  j_bit2/1 -> Subsystem2/2(j_bit)
  Subsystem2/1(din_sel) -> wr_sel_2/1
  Subsystem/1(din_sel) -> wr_sel_0/1
  i_bit3/1 -> Subsystem3/1(i_bit)
  Subsystem/2(en) -> wr_en_0/1
  i_bit0/1 -> Subsystem/1(i_bit)
  Subsystem3/2(en) -> wr_en_3/1
  j_bit0/1 -> Subsystem/2(j_bit)
  Subsystem4/1(din_sel) -> wr_sel_4/1
  i_bit1/1 -> Subsystem1/1(i_bit)

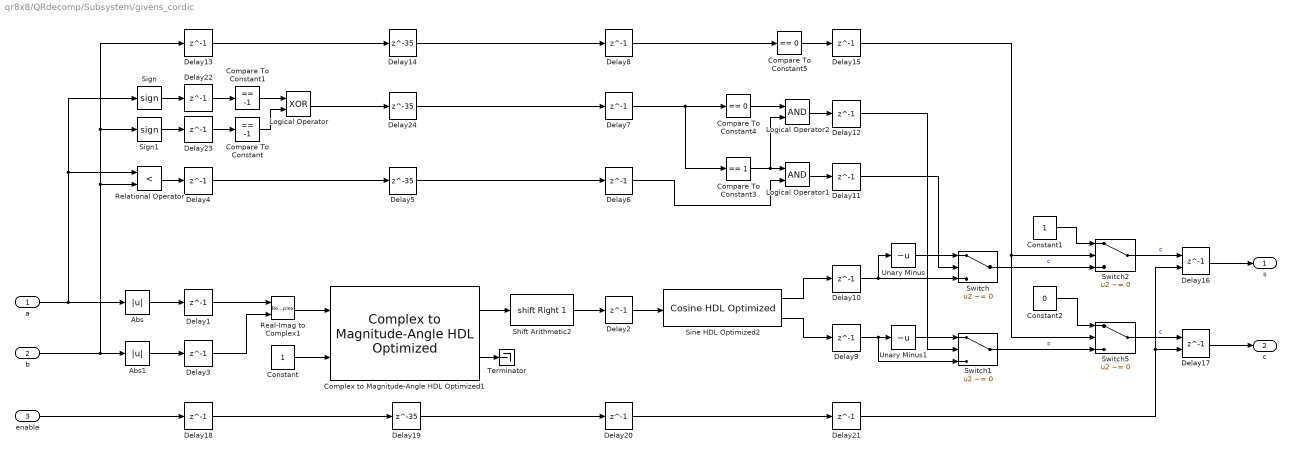
== system qr8x8/QRdecomp/Subsystem/givens_cordic ==
  a : Inport
  b : Inport  Port=2
  enable : Inport  Port=3
  Abs : Abs
  Abs1 : Abs
  Compare To Constant : simulink/Logic and Bit Operations/Compare To Constant  relop===  const=-1  OutDataTypeStr=boolean
  Compare To Constant1 : simulink/Logic and Bit Operations/Compare To Constant  relop===  const=-1  OutDataTypeStr=boolean
  Compare To Constant3 : simulink/Logic and Bit Operations/Compare To Constant  relop===  const=1  OutDataTypeStr=boolean
  Compare To Constant4 : simulink/Logic and Bit Operations/Compare To Constant  relop===  const=0  OutDataTypeStr=boolean
  Compare To Constant5 : simulink/Logic and Bit Operations/Compare To Constant  relop===  const=0  OutDataTypeStr=boolean
  Complex to Magnitude-Angle HDL Optimized1 : dspmathops/Complex to Magnitude-Angle HDL Optimized  NumIterationsSource=Auto  NumIterations=8  OutputFormat=Angle  AngleFormat=Normalized  ScaleOutput=on  SimulateUsing=Code generation
      settings: SourceProductName=DSP System Toolbox  SourceProductBaseCode=DS
  Constant : Constant  OutDataTypeStr=boolean  SampleTime=-1
  Constant1 : Constant  OutDataTypeStr=fixdt(1,32,30)  SampleTime=-1
  Constant2 : Constant  Value=0  OutDataTypeStr=fixdt(1,32,30)  SampleTime=-1
  Delay{1..4,6..13,15,18,20..23} (18 alike) : Delay  DelayLength=1
  Delay{5,14,19,24} (4 alike) : Delay  DelayLength=35
  Delay16 : Delay  DelayLength=1  ShowEnablePort=on
      settings: InputPortMap=u0,e6
  Delay17 : Delay  DelayLength=1  ShowEnablePort=on
      settings: InputPortMap=u0,e6
  Logical Operator : Logic  Operator=XOR  AllPortsSameDT=off  OutDataTypeStr=boolean
  Logical Operator1 : Logic  AllPortsSameDT=off  OutDataTypeStr=boolean
  Logical Operator2 : Logic  AllPortsSameDT=off  OutDataTypeStr=boolean
  Real-Imag to Complex1 : RealImagToComplex
  Relational Operator : RelationalOperator  Operator=<  OutDataTypeStr=boolean  RndMeth=Nearest
  Shift Arithmetic2 : ArithShift  BitShiftNumber=1  BitShiftDirection=Right
  Sign : Signum
  Sign1 : Signum
  Sine HDL Optimized2 : hdlsllib/Lookup Tables/Cosine HDL Optimized  OutputFormula=sin(2*pi*u) and cos(2*pi*u)  NumDataPoints=512  TableDataTypeStr=fixdt(1,32,30)  SimulateLUTROMDelay=off
      settings: SourceProductName=HDL Coder  SourceProductBaseCode=HD
  Switch{,1..2,5} (4 alike) : Switch  Criteria=u2 ~= 0
  Terminator : Terminator
  Unary Minus : UnaryMinus
  Unary Minus1 : UnaryMinus
  s : Outport
  c : Outport  Port=2
  wires:
  Delay2/1 -> Sine HDL Optimized2/1
  Shift Arithmetic2/1 -> Delay2/1
  Real-Imag to Complex1/1 -> Complex to Magnitude-Angle HDL Optimized1/1
  Complex to Magnitude-Angle HDL Optimized1/2 -> Terminator/1
  Constant/1 -> Complex to Magnitude-Angle HDL Optimized1/2
  Complex to Magnitude-Angle HDL Optimized1/1 -> Shift Arithmetic2/1
  Sine HDL Optimized2/1 -> Delay10/1
  Sine HDL Optimized2/2 -> Delay9/1
  Abs/1 -> Delay1/1
  Abs1/1 -> Delay3/1
  Compare To Constant3/1 -> Logical Operator2/2, Logical Operator1/1
  Delay23/1 -> Compare To Constant/1
  Delay13/1 -> Delay14/1
  Sign/1 -> Delay22/1
  Compare To Constant4/1 -> Logical Operator2/1
  Compare To Constant1/1 -> Logical Operator/1
  Delay22/1 -> Compare To Constant1/1
  Compare To Constant/1 -> Logical Operator/2
  Logical Operator/1 -> Delay24/1
  Sign1/1 -> Delay23/1
  Delay16/1 -> s/1
  Switch5/1 -> Delay17/1  "c"
  Switch/1 -> Switch2/3  "c"
  Constant2/1 -> Switch5/1
  Constant1/1 -> Switch2/1
  Switch1/1 -> Switch5/3  "s"
  Switch2/1 -> Delay16/1  "c"
  Delay17/1 -> c/1
  Delay1/1 -> Real-Imag to Complex1/1
  Delay3/1 -> Real-Imag to Complex1/2
  b/1 -> Relational Operator/2, Delay13/1, Sign1/1, Abs1/1
  a/1 -> Relational Operator/1, Sign/1, Abs/1
  Relational Operator/1 -> Delay4/1
  Delay4/1 -> Delay5/1
  Delay5/1 -> Delay6/1
  Delay24/1 -> Delay7/1
  Delay14/1 -> Delay8/1
  Delay7/1 -> Compare To Constant3/1, Compare To Constant4/1
  Delay6/1 -> Logical Operator1/2
  Unary Minus/1 -> Switch/1
  Unary Minus1/1 -> Switch1/1
  Logical Operator1/1 -> Delay11/1
  Logical Operator2/1 -> Delay12/1
  Delay8/1 -> Compare To Constant5/1
  Compare To Constant5/1 -> Delay15/1
  Delay19/1 -> Delay20/1
  Delay21/1 -> Delay17/2, Delay16/2
  Delay20/1 -> Delay21/1
  Delay18/1 -> Delay19/1
  enable/1 -> Delay18/1
  Delay9/1 -> Switch1/3, Unary Minus1/1
  Delay10/1 -> Unary Minus/1, Switch/3
  Delay11/1 -> Switch/2
  Delay12/1 -> Switch1/2
  Delay15/1 -> Switch5/2, Switch2/2

== system qr8x8/QRdecomp/Subsystem/trig1 ==
  trigger : Inport
  Compare To Constant2 : simulink/Logic and Bit Operations/Compare To Constant  relop===  const=2  OutDataTypeStr=boolean
  Compare To Constant3 : simulink/Logic and Bit Operations/Compare To Constant  relop===  const=0  OutDataTypeStr=boolean
  Constant : Constant  OutDataTypeStr=boolean  SampleTime=-1
  Enabled Resettable Delay : Delay  DelayLength=1  ExternalReset=Level
      settings: InputPortMap=u0,r5
  HDL Counter : hdlsllib/Sources/HDL Counter  CountType=Count limited  CountInit=0  CountStep=1  CountMax=2  CountFromType=Initial value  CountFrom=0  CountResetPort=on  CountLoadPort=off  CountEnbPort=on  CountDirPort=off  CountDataType=Unsigned  CountWordLen=4  CountFracLen=0  CountSampTime=1
      settings: SourceProductBaseCode=HD
  Switch : Switch  Criteria=u2 ~= 0
  en : Outport
  wires:
  Compare To Constant2/1 -> Enabled Resettable Delay/2
  Enabled Resettable Delay/1 -> Switch/3, Compare To Constant3/1, HDL Counter/2, en/1
  Compare To Constant3/1 -> HDL Counter/1
  HDL Counter/1 -> Compare To Constant2/1
  Switch/1 -> Enabled Resettable Delay/1
  Constant/1 -> Switch/1
  trigger/1 -> Switch/2

== system qr8x8/QRdecomp/Q_col/Subsystem/Subsystem ==
  sel : Inport
  load : Inport  Port=2
  din_i : Inport  Port=3
  "din_j " : Inport  Port=4
  din_load : Inport  Port=5
  Bit Slice : hdlsllib/Logic and Bit Operations/Bit Slice  lidx=1  ridx=1
  Bit Slice1 : hdlsllib/Logic and Bit Operations/Bit Slice  lidx=0  ridx=0
  Constant : Constant  Value=0  OutDataTypeStr=fixdt(1,32,25)  SampleTime=-1
  Logical Operator : Logic  Operator=XOR  AllPortsSameDT=off  OutDataTypeStr=boolean
  Switch : Switch  Criteria=u2 ~= 0
  Switch1 : Switch  Criteria=u2 ~= 0
  Switch2 : Switch  Criteria=u2 ~= 0
  din : Outport
  wires:
  Constant/1 -> Switch2/3
  Logical Operator/1 -> Switch2/2
  sel/1 -> Bit Slice1/1, Bit Slice/1
  din_i/1 -> Switch/1
  Bit Slice1/1 -> Switch/2, Logical Operator/2
  Bit Slice/1 -> Logical Operator/1
  Switch/1 -> Switch2/1
  "din_j "/1 -> Switch/3
  Switch1/1 -> din/1
  din_load/1 -> Switch1/1
  load/1 -> Switch1/2
  Switch2/1 -> Switch1/3

== system qr8x8/QRdecomp/Q_col/Subsystem/Subsystem1 ==
  sel : Inport
  load : Inport  Port=2
  din_i : Inport  Port=3
  "din_j " : Inport  Port=4
  din_load : Inport  Port=5
  Bit Slice : hdlsllib/Logic and Bit Operations/Bit Slice  lidx=1  ridx=1
  Bit Slice1 : hdlsllib/Logic and Bit Operations/Bit Slice  lidx=0  ridx=0
  Constant : Constant  Value=0  OutDataTypeStr=fixdt(1,32,25)  SampleTime=-1
  Logical Operator : Logic  Operator=XOR  AllPortsSameDT=off  OutDataTypeStr=boolean
  Switch : Switch  Criteria=u2 ~= 0
  Switch1 : Switch  Criteria=u2 ~= 0
  Switch2 : Switch  Criteria=u2 ~= 0
  din : Outport
  wires:
  Switch2/1 -> Switch1/3
  load/1 -> Switch1/2
  din_load/1 -> Switch1/1
  Switch1/1 -> din/1
  "din_j "/1 -> Switch/3
  Switch/1 -> Switch2/1
  Bit Slice/1 -> Logical Operator/1
  Bit Slice1/1 -> Logical Operator/2, Switch/2
  din_i/1 -> Switch/1
  sel/1 -> Bit Slice/1, Bit Slice1/1
  Logical Operator/1 -> Switch2/2
  Constant/1 -> Switch2/3

== system qr8x8/QRdecomp/Q_col/Subsystem/Subsystem2 ==
  sel : Inport
  load : Inport  Port=2
  din_i : Inport  Port=3
  "din_j " : Inport  Port=4
  din_load : Inport  Port=5
  Bit Slice : hdlsllib/Logic and Bit Operations/Bit Slice  lidx=1  ridx=1
  Bit Slice1 : hdlsllib/Logic and Bit Operations/Bit Slice  lidx=0  ridx=0
  Constant1 : Constant  Value=0  OutDataTypeStr=fixdt(1,32,25)  SampleTime=-1
  Logical Operator : Logic  Operator=XOR  AllPortsSameDT=off  OutDataTypeStr=boolean
  Switch : Switch  Criteria=u2 ~= 0
  Switch1 : Switch  Criteria=u2 ~= 0
  Switch2 : Switch  Criteria=u2 ~= 0
  din : Outport
  wires:
  Constant1/1 -> Switch2/3
  Logical Operator/1 -> Switch2/2
  sel/1 -> Bit Slice1/1, Bit Slice/1
  din_i/1 -> Switch/1
  Bit Slice1/1 -> Switch/2, Logical Operator/2
  Bit Slice/1 -> Logical Operator/1
  Switch/1 -> Switch2/1
  "din_j "/1 -> Switch/3
  Switch1/1 -> din/1
  din_load/1 -> Switch1/1
  load/1 -> Switch1/2
  Switch2/1 -> Switch1/3

== system qr8x8/QRdecomp/Q_col/Subsystem/Subsystem3 ==
  sel : Inport
  load : Inport  Port=2
  din_i : Inport  Port=3
  "din_j " : Inport  Port=4
  din_load : Inport  Port=5
  Bit Slice : hdlsllib/Logic and Bit Operations/Bit Slice  lidx=1  ridx=1
  Bit Slice1 : hdlsllib/Logic and Bit Operations/Bit Slice  lidx=0  ridx=0
  Constant : Constant  Value=0  OutDataTypeStr=fixdt(1,32,25)  SampleTime=-1
  Logical Operator : Logic  Operator=XOR  AllPortsSameDT=off  OutDataTypeStr=boolean
  Switch : Switch  Criteria=u2 ~= 0
  Switch1 : Switch  Criteria=u2 ~= 0
  Switch2 : Switch  Criteria=u2 ~= 0
  din : Outport
  wires:
  Switch2/1 -> Switch1/3
  load/1 -> Switch1/2
  din_load/1 -> Switch1/1
  Switch1/1 -> din/1
  "din_j "/1 -> Switch/3
  Switch/1 -> Switch2/1
  Bit Slice/1 -> Logical Operator/1
  Bit Slice1/1 -> Logical Operator/2, Switch/2
  din_i/1 -> Switch/1
  sel/1 -> Bit Slice/1, Bit Slice1/1
  Logical Operator/1 -> Switch2/2
  Constant/1 -> Switch2/3

== system qr8x8/QRdecomp/Q_col/Subsystem/Subsystem4 ==
  sel : Inport
  load : Inport  Port=2
  din_i : Inport  Port=3
  "din_j " : Inport  Port=4
  din_load : Inport  Port=5
  Bit Slice : hdlsllib/Logic and Bit Operations/Bit Slice  lidx=1  ridx=1
  Bit Slice1 : hdlsllib/Logic and Bit Operations/Bit Slice  lidx=0  ridx=0
  Constant : Constant  Value=0  OutDataTypeStr=fixdt(1,32,25)  SampleTime=-1
  Logical Operator : Logic  Operator=XOR  AllPortsSameDT=off  OutDataTypeStr=boolean
  Switch : Switch  Criteria=u2 ~= 0
  Switch1 : Switch  Criteria=u2 ~= 0
  Switch2 : Switch  Criteria=u2 ~= 0
  din : Outport
  wires:
  Constant/1 -> Switch2/3
  Logical Operator/1 -> Switch2/2
  sel/1 -> Bit Slice1/1, Bit Slice/1
  din_i/1 -> Switch/1
  Bit Slice1/1 -> Switch/2, Logical Operator/2
  Bit Slice/1 -> Logical Operator/1
  Switch/1 -> Switch2/1
  "din_j "/1 -> Switch/3
  Switch1/1 -> din/1
  din_load/1 -> Switch1/1
  load/1 -> Switch1/2
  Switch2/1 -> Switch1/3

== system qr8x8/QRdecomp/Q_col/Subsystem/Subsystem5 ==
  sel : Inport
  load : Inport  Port=2
  din_i : Inport  Port=3
  "din_j " : Inport  Port=4
  din_load : Inport  Port=5
  Bit Slice : hdlsllib/Logic and Bit Operations/Bit Slice  lidx=1  ridx=1
  Bit Slice1 : hdlsllib/Logic and Bit Operations/Bit Slice  lidx=0  ridx=0
  Constant : Constant  Value=0  OutDataTypeStr=fixdt(1,32,25)  SampleTime=-1
  Logical Operator : Logic  Operator=XOR  AllPortsSameDT=off  OutDataTypeStr=boolean
  Switch : Switch  Criteria=u2 ~= 0
  Switch1 : Switch  Criteria=u2 ~= 0
  Switch2 : Switch  Criteria=u2 ~= 0
  din : Outport
  wires:
  Switch2/1 -> Switch1/3
  load/1 -> Switch1/2
  din_load/1 -> Switch1/1
  Switch1/1 -> din/1
  "din_j "/1 -> Switch/3
  Switch/1 -> Switch2/1
  Bit Slice/1 -> Logical Operator/1
  Bit Slice1/1 -> Logical Operator/2, Switch/2
  din_i/1 -> Switch/1
  sel/1 -> Bit Slice/1, Bit Slice1/1
  Logical Operator/1 -> Switch2/2
  Constant/1 -> Switch2/3

== system qr8x8/QRdecomp/Q_col/Subsystem/Subsystem6 ==
  sel : Inport
  load : Inport  Port=2
  din_i : Inport  Port=3
  "din_j " : Inport  Port=4
  din_load : Inport  Port=5
  Bit Slice : hdlsllib/Logic and Bit Operations/Bit Slice  lidx=1  ridx=1
  Bit Slice1 : hdlsllib/Logic and Bit Operations/Bit Slice  lidx=0  ridx=0
  Constant : Constant  Value=0  OutDataTypeStr=fixdt(1,32,25)  SampleTime=-1
  Logical Operator : Logic  Operator=XOR  AllPortsSameDT=off  OutDataTypeStr=boolean
  Switch : Switch  Criteria=u2 ~= 0
  Switch1 : Switch  Criteria=u2 ~= 0
  Switch2 : Switch  Criteria=u2 ~= 0
  din : Outport
  wires:
  Constant/1 -> Switch2/3
  Logical Operator/1 -> Switch2/2
  sel/1 -> Bit Slice1/1, Bit Slice/1
  din_i/1 -> Switch/1
  Bit Slice1/1 -> Switch/2, Logical Operator/2
  Bit Slice/1 -> Logical Operator/1
  Switch/1 -> Switch2/1
  "din_j "/1 -> Switch/3
  Switch1/1 -> din/1
  din_load/1 -> Switch1/1
  load/1 -> Switch1/2
  Switch2/1 -> Switch1/3

== system qr8x8/QRdecomp/Q_col/Subsystem/Subsystem7 ==
  sel : Inport
  load : Inport  Port=2
  din_i : Inport  Port=3
  "din_j " : Inport  Port=4
  din_load : Inport  Port=5
  Bit Slice : hdlsllib/Logic and Bit Operations/Bit Slice  lidx=1  ridx=1
  Bit Slice1 : hdlsllib/Logic and Bit Operations/Bit Slice  lidx=0  ridx=0
  Constant : Constant  Value=0  OutDataTypeStr=fixdt(1,32,25)  SampleTime=-1
  Logical Operator : Logic  Operator=XOR  AllPortsSameDT=off  OutDataTypeStr=boolean
  Switch : Switch  Criteria=u2 ~= 0
  Switch1 : Switch  Criteria=u2 ~= 0
  Switch2 : Switch  Criteria=u2 ~= 0
  din : Outport
  wires:
  Switch2/1 -> Switch1/3
  load/1 -> Switch1/2
  din_load/1 -> Switch1/1
  Switch1/1 -> din/1
  "din_j "/1 -> Switch/3
  Switch/1 -> Switch2/1
  Bit Slice/1 -> Logical Operator/1
  Bit Slice1/1 -> Logical Operator/2, Switch/2
  din_i/1 -> Switch/1
  sel/1 -> Bit Slice/1, Bit Slice1/1
  Logical Operator/1 -> Switch2/2
  Constant/1 -> Switch2/3

== system qr8x8/QRdecomp/Q_col/Subsystem5/Subsystem ==
  i_bit : Inport
  j_bit : Inport  Port=2
  load : Inport  Port=3
  wr_en : Inport  Port=4
  Bit Concat : hdlsllib/Logic and Bit Operations/Bit Concat  numInputs=2
      settings: SourceProductName=HDL Coder  SourceProductBaseCode=HD
  Logical Operator : Logic  Operator=OR  AllPortsSameDT=off  OutDataTypeStr=boolean
  Logical Operator1 : Logic  Operator=OR  AllPortsSameDT=off  OutDataTypeStr=boolean
  Logical Operator2 : Logic  AllPortsSameDT=off  OutDataTypeStr=boolean
  din_sel : Outport
  en : Outport  Port=2
  wires:
  j_bit/1 -> Logical Operator/2, Bit Concat/1
  Bit Concat/1 -> din_sel/1
  Logical Operator/1 -> Logical Operator1/1
  load/1 -> Logical Operator1/2
  Logical Operator1/1 -> Logical Operator2/1
  wr_en/1 -> Logical Operator2/2
  Logical Operator2/1 -> en/1
  i_bit/1 -> Bit Concat/2, Logical Operator/1

== system qr8x8/QRdecomp/Q_col/Subsystem5/Subsystem1 ==
  i_bit : Inport
  j_bit : Inport  Port=2
  load : Inport  Port=3
  wr_en : Inport  Port=4
  Bit Concat : hdlsllib/Logic and Bit Operations/Bit Concat  numInputs=2
      settings: SourceProductName=HDL Coder  SourceProductBaseCode=HD
  Logical Operator : Logic  Operator=OR  AllPortsSameDT=off  OutDataTypeStr=boolean
  Logical Operator1 : Logic  Operator=OR  AllPortsSameDT=off  OutDataTypeStr=boolean
  Logical Operator2 : Logic  AllPortsSameDT=off  OutDataTypeStr=boolean
  din_sel : Outport
  en : Outport  Port=2
  wires:
  i_bit/1 -> Logical Operator/1, Bit Concat/2
  Logical Operator2/1 -> en/1
  wr_en/1 -> Logical Operator2/2
  Logical Operator1/1 -> Logical Operator2/1
  load/1 -> Logical Operator1/2
  Logical Operator/1 -> Logical Operator1/1
  Bit Concat/1 -> din_sel/1
  j_bit/1 -> Bit Concat/1, Logical Operator/2

== system qr8x8/QRdecomp/Q_col/Subsystem5/Subsystem2 ==
  i_bit : Inport
  j_bit : Inport  Port=2
  load : Inport  Port=3
  wr_en : Inport  Port=4
  Bit Concat : hdlsllib/Logic and Bit Operations/Bit Concat  numInputs=2
      settings: SourceProductName=HDL Coder  SourceProductBaseCode=HD
  Logical Operator : Logic  Operator=OR  AllPortsSameDT=off  OutDataTypeStr=boolean
  Logical Operator1 : Logic  Operator=OR  AllPortsSameDT=off  OutDataTypeStr=boolean
  Logical Operator2 : Logic  AllPortsSameDT=off  OutDataTypeStr=boolean
  din_sel : Outport
  en : Outport  Port=2
  wires:
  j_bit/1 -> Logical Operator/2, Bit Concat/1
  Bit Concat/1 -> din_sel/1
  Logical Operator/1 -> Logical Operator1/1
  load/1 -> Logical Operator1/2
  Logical Operator1/1 -> Logical Operator2/1
  wr_en/1 -> Logical Operator2/2
  Logical Operator2/1 -> en/1
  i_bit/1 -> Bit Concat/2, Logical Operator/1

== system qr8x8/QRdecomp/Q_col/Subsystem5/Subsystem3 ==
  i_bit : Inport
  j_bit : Inport  Port=2
  load : Inport  Port=3
  wr_en : Inport  Port=4
  Bit Concat : hdlsllib/Logic and Bit Operations/Bit Concat  numInputs=2
      settings: SourceProductName=HDL Coder  SourceProductBaseCode=HD
  Logical Operator : Logic  Operator=OR  AllPortsSameDT=off  OutDataTypeStr=boolean
  Logical Operator1 : Logic  Operator=OR  AllPortsSameDT=off  OutDataTypeStr=boolean
  Logical Operator2 : Logic  AllPortsSameDT=off  OutDataTypeStr=boolean
  din_sel : Outport
  en : Outport  Port=2
  wires:
  i_bit/1 -> Logical Operator/1, Bit Concat/2
  Logical Operator2/1 -> en/1
  wr_en/1 -> Logical Operator2/2
  Logical Operator1/1 -> Logical Operator2/1
  load/1 -> Logical Operator1/2
  Logical Operator/1 -> Logical Operator1/1
  Bit Concat/1 -> din_sel/1
  j_bit/1 -> Bit Concat/1, Logical Operator/2

== system qr8x8/QRdecomp/Q_col/Subsystem5/Subsystem4 ==
  i_bit : Inport
  j_bit : Inport  Port=2
  load : Inport  Port=3
  wr_en : Inport  Port=4
  Bit Concat : hdlsllib/Logic and Bit Operations/Bit Concat  numInputs=2
      settings: SourceProductName=HDL Coder  SourceProductBaseCode=HD
  Logical Operator : Logic  Operator=OR  AllPortsSameDT=off  OutDataTypeStr=boolean
  Logical Operator1 : Logic  Operator=OR  AllPortsSameDT=off  OutDataTypeStr=boolean
  Logical Operator2 : Logic  AllPortsSameDT=off  OutDataTypeStr=boolean
  din_sel : Outport
  en : Outport  Port=2
  wires:
  j_bit/1 -> Logical Operator/2, Bit Concat/1
  Bit Concat/1 -> din_sel/1
  Logical Operator/1 -> Logical Operator1/1
  load/1 -> Logical Operator1/2
  Logical Operator1/1 -> Logical Operator2/1
  wr_en/1 -> Logical Operator2/2
  Logical Operator2/1 -> en/1
  i_bit/1 -> Bit Concat/2, Logical Operator/1
